simulink model "gm_sampleModel1706_1_sub"  (R2023a)
settings: Solver=VariableStepAuto  StartTime=0.0  StopTime=10.0  RelTol=1e-3
libraries: simulink x4
settings Model: Creator=user1  LastModifiedBy=user1
settings OptimizationCC: BlockReduction=off  ConditionallyExecuteInputs=off
settings DebuggingCC: InheritedTsInSrcMsg=none

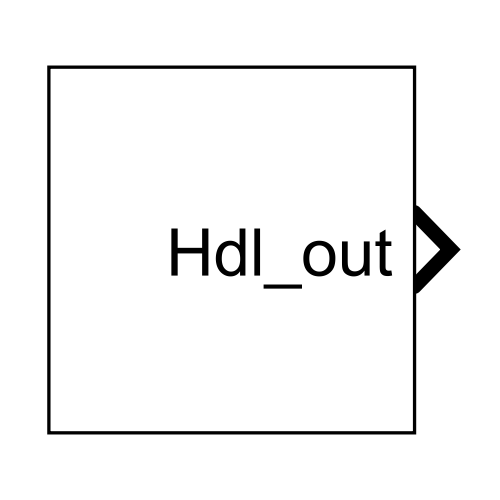
[thumbnail: Simulink's stored preview of the top-level diagram]
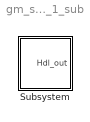
== system gm_sampleModel1706_1_sub ==
  Subsystem : Subsystem

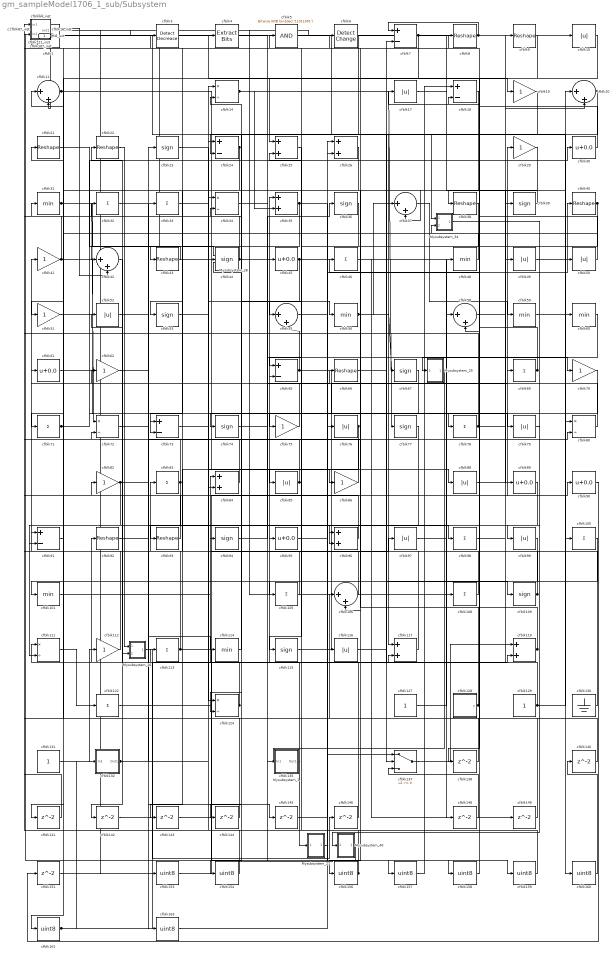
== system gm_sampleModel1706_1_sub/Subsystem ==
  Mysubsystem_1 : Subsystem
  Mysubsystem_25 : Subsystem
  Mysubsystem_26 : Subsystem
  Mysubsystem_27 : Subsystem
  Mysubsystem_28 : Subsystem
  Mysubsystem_34 : Subsystem
  Mysubsystem_40 : Subsystem
  cfblk1 : Logic  AllPortsSameDT=off  OutDataTypeStr=boolean
  cfblk{10,17,49..50,52,76,79,85,88,97,99,116} (12 alike) : Abs  OutDataTypeStr=uint8  SaturateOnIntegerOverflow=off
  cfblk{32..33,46,69,71,78,83,98,100,105,108,113,122} (13 alike) : Sum  Inputs=+  OutDataTypeStr=uint8
  cfblk{31,48,56,59..60,101,114} (7 alike) : MinMax  OutDataTypeStr=uint8
  cfblk103_inst : Subsystem
  cfblk{11,20,37,42,55,58,106} (7 alike) : Sum  Inputs=|++  OutDataTypeStr=uint8
  cfblk107_inst : Subsystem
  cfblk{23,36,39,44,53,67,74,77,94,109,115} (11 alike) : Signum
  cfblk{14,34,72,80,111,124} (6 alike) : Product  Inputs=*/  OutDataTypeStr=uint8  RndMeth=Zero  SaturateOnIntegerOverflow=on
  cfblk{19,29,41,51,62,70,75,82,86,112} (10 alike) : Gain  OutDataTypeStr=uint8
  cfblk{25..26,35,84,96,117,119} (7 alike) : Sum  OutDataTypeStr=uint8
  cfblk121_inst : Subsystem
  cfblk127 : Constant  OutDataTypeStr=uint8  SampleTime=-1
  cfblk128 : Subsystem  mask(Counter Limited){uplimit=double(7), tsamp=double(-1)}
      mask prompts: uplimit "Simulink:masks:UpperLimit_MP"; tsamp "Simulink:masks:SampleTime_MP"
      mask help: Simulink:masks:CounterLimited_MD
      mask init:
      | nbits = double(8);
      | tsamp = double(-1);
      | uplimit = double(7);
  cfblk129 : Constant  OutDataTypeStr=uint8  SampleTime=-1
  cfblk130 : Ground
  cfblk131 : Constant  OutDataTypeStr=uint8  SampleTime=-1
  cfblk132 : Subsystem
  cfblk135 : Subsystem
  cfblk137 : Switch  OutDataTypeStr=uint8  SaturateOnIntegerOverflow=off  InputSameDT=off
  cfblk{138,140..146,148..149,151} (11 alike) : Delay  SampleTime=1
  cfblk{153..154,156..161,163} (9 alike) : DataTypeConversion  OutDataTypeStr=uint8  SaturateOnIntegerOverflow=off  RndMeth=Floor
  cfblk16_inst : Subsystem
  cfblk{7,18,24,65,73,91} (6 alike) : Sum  Inputs=+-  OutDataTypeStr=uint8
  cfblk2 : Constant  Value=0  OutDataTypeStr=uint8  SampleTime=1
  cfblk{8..9,21..22,38,40,43,66,92..93} (10 alike) : Reshape
  cfblk3 : simulink/Logic and Bit Operations/Detect Decrease  vinit=0.0  OutDataTypeStr=uint8
      settings: LibrarySourceBlock=|
      | hdlsllib/Logic and Bit
      | Operations/Detect
      | Decrease
  cfblk{30,45,61,89..90,95} (6 alike) : Bias  Bias=0.0  SaturateOnIntegerOverflow=off
  cfblk4 : simulink/Logic and Bit Operations/Extract Bits  bitsToExtract=Upper half  numBits=8  bitIdxRange=[0 7]  outScalingMode=Preserve fixed-point scaling
      settings: LibrarySourceBlock=|
      | hdlsllib/Logic and Bit
      | Operations/Extract Bits
  cfblk5 : simulink/Logic and Bit Operations/Bitwise Operator  logicop=AND  UseBitMask=on  BitMask=bin2dec('11011001')  BitMaskRealWorld=Stored Integer
      settings: LibrarySourceBlock=|
      | hdlsllib/Logic and Bit
      | Operations/Bitwise
      | Operator
  cfblk6 : simulink/Logic and Bit Operations/Detect Change  vinit=0  OutDataTypeStr=uint8
      settings: LibrarySourceBlock=|
      | hdlsllib/Logic and Bit
      | Operations/Detect
      | Change
  cfblk64_inst : Subsystem
  cfblk87_inst : Subsystem
  Hdl_out : Outport  OutDataTypeStr=uint8  SampleTime=1
  wires:
  Mysubsystem_1/1(Out1) -> Mysubsystem_27/1(In1)
  Mysubsystem_25/1(Out1) -> Mysubsystem_1/1(In1)
  Mysubsystem_26/1(Out1) -> cfblk146/1
  Mysubsystem_27/1(Out1) -> cfblk26/1
  Mysubsystem_28/1(Out1) -> cfblk149/1
  Mysubsystem_34/1(Out1) -> Mysubsystem_40/1(In1)
  Mysubsystem_40/1(Out1) -> cfblk64_inst/2(in2)
  cfblk1/1 -> cfblk117/1
  cfblk10/1 -> cfblk25/1
  cfblk100/1 -> cfblk101/1
  cfblk101/1 -> cfblk84/1
  cfblk103_inst/1(out1) -> cfblk4/1
  cfblk105/1 -> cfblk35/1
  cfblk106/1 -> cfblk41/1
  cfblk107_inst/1(out1) -> cfblk45/1, cfblk33/1
  cfblk108/1 -> cfblk103_inst/1(in1)
  cfblk109/1 -> cfblk58/2, Mysubsystem_28/2(In2)
  cfblk11/1 -> cfblk88/1, cfblk71/1
  cfblk111/1 -> cfblk122/1
  cfblk112/1 -> cfblk121_inst/1(in1)
  cfblk113/1 -> cfblk91/1, cfblk158/1, cfblk29/1
  cfblk114/1 -> cfblk34/2
  cfblk115/1 -> cfblk69/1
  cfblk116/1 -> cfblk90/1
  cfblk117/1 -> cfblk3/1
  cfblk119/1 -> cfblk38/1, cfblk103_inst/2(in2)
  cfblk121_inst/1(out1) -> cfblk10/1
  cfblk122/1 -> cfblk97/1
  cfblk124/1 -> cfblk92/1, cfblk22/1
  cfblk127/1 -> cfblk58/1
  cfblk128/1(y) -> cfblk72/2, cfblk113/1
  cfblk129/1 -> cfblk20/1, cfblk111/1
  cfblk130/1 -> cfblk83/1
  cfblk131/1 -> cfblk112/1
  cfblk132/1(Out1) -> cfblk44/1, cfblk23/1
  cfblk135/1(Out1) -> cfblk94/1
  cfblk137/1 -> cfblk119/1
  cfblk138/1 -> cfblk1/1
  cfblk14/1 -> cfblk77/1, cfblk35/2
  cfblk140/1 -> cfblk107_inst/1(in1)
  cfblk141/1 -> cfblk87_inst/1(in1)
  cfblk142/1 -> cfblk7/2
  cfblk143/1 -> cfblk117/2
  cfblk144/1 -> cfblk1/2
  cfblk145/1 -> cfblk137/1
  cfblk146/1 -> cfblk65/2
  cfblk148/1 -> cfblk137/3
  cfblk149/1 -> cfblk106/1
  cfblk151/1 -> cfblk119/2
  cfblk153/1 -> cfblk95/1
  cfblk154/1 -> cfblk64_inst/1(in1)
  cfblk156/1 -> cfblk87_inst/2(in2), cfblk34/1
  cfblk157/1 -> cfblk18/1
  cfblk158/1 -> cfblk18/2
  cfblk159/1 -> cfblk5/1
  cfblk16_inst/1(out1) -> cfblk108/1
  cfblk160/1 -> cfblk140/1
  cfblk161/1 -> cfblk9/1, cfblk132/1(In1)
  cfblk163/1 -> cfblk26/2
  cfblk17/1 -> cfblk100/1
  cfblk18/1 -> cfblk156/1
  cfblk19/1 -> cfblk137/2
  cfblk2/1 -> cfblk42/2
  cfblk20/1 -> cfblk24/2, Mysubsystem_34/1(In1)
  cfblk21/1 -> cfblk43/1
  cfblk22/1 -> Mysubsystem_26/1(In1)
  cfblk23/1 -> cfblk86/1
  cfblk24/1 -> cfblk53/1, cfblk141/1
  cfblk25/1 -> cfblk85/1
  cfblk26/1 -> cfblk161/1
  cfblk29/1 -> cfblk84/2
  cfblk3/1 -> cfblk19/1
  cfblk30/1 -> cfblk8/1
  cfblk31/1 -> cfblk72/1, Mysubsystem_28/1(In1)
  cfblk32/1 -> cfblk96/2
  cfblk33/1 -> cfblk56/1
  cfblk34/1 -> cfblk159/1
  cfblk35/1 -> cfblk76/1, cfblk73/2
  cfblk36/1 -> cfblk55/1
  cfblk37/1 -> cfblk59/1
  cfblk38/1 -> cfblk65/1
  cfblk39/1 -> cfblk37/2
  cfblk4/1 -> cfblk96/1
  cfblk40/1 -> cfblk75/1, Mysubsystem_34/2(In2)
  cfblk41/1 -> cfblk135/1(In1), cfblk31/1
  cfblk42/1 -> cfblk142/1
  cfblk43/1 -> cfblk42/1
  cfblk44/1 -> cfblk107_inst/2(in2), cfblk70/1
  cfblk45/1 -> cfblk25/2, cfblk124/2
  cfblk46/1 -> cfblk148/1
  cfblk48/1 -> cfblk11/1
  cfblk49/1 -> cfblk40/1
  cfblk5/1 -> cfblk160/1
  cfblk50/1 -> cfblk17/1
  cfblk51/1 -> cfblk78/1
  cfblk52/1 -> cfblk114/1
  cfblk53/1 -> cfblk14/1
  cfblk55/1 -> cfblk50/1
  cfblk56/1 -> cfblk67/1, cfblk37/1
  cfblk58/1 -> cfblk20/2
  cfblk59/1 -> cfblk60/1
  cfblk6/1 -> cfblk154/1
  cfblk60/1 -> Mysubsystem_25/1(In1)
  cfblk61/1 -> cfblk116/1
  cfblk62/1 -> cfblk163/1
  cfblk64_inst/1(out1) -> cfblk153/1
  cfblk65/1 -> cfblk79/1, cfblk55/2
  cfblk66/1 -> cfblk109/1
  cfblk67/1 -> cfblk115/1
  cfblk69/1 -> cfblk6/1, cfblk46/1
  cfblk7/1 -> cfblk89/1, cfblk51/1
  cfblk70/1 -> cfblk74/1
  cfblk71/1 -> cfblk73/1, cfblk30/1
  cfblk72/1 -> cfblk98/1
  cfblk73/1 -> cfblk124/1
  cfblk74/1 -> cfblk66/1
  cfblk75/1 -> cfblk24/1
  cfblk76/1 -> cfblk144/1, cfblk143/1
  cfblk77/1 -> cfblk91/2
  cfblk78/1 -> cfblk49/1, cfblk16_inst/1(in1), cfblk14/2
  cfblk79/1 -> cfblk99/1
  cfblk8/1 -> cfblk7/1, Hdl_out/1
  cfblk80/1 -> cfblk61/1
  cfblk82/1 -> cfblk80/2, cfblk111/2
  cfblk83/1 -> cfblk93/1, cfblk16_inst/2(in2)
  cfblk84/1 -> cfblk62/1
  cfblk85/1 -> cfblk52/1, cfblk105/1
  cfblk86/1 -> cfblk32/1
  cfblk87_inst/1(out1) -> cfblk11/2
  cfblk88/1 -> cfblk39/1
  cfblk89/1 -> Mysubsystem_26/2(In2)
  cfblk9/1 -> cfblk138/1
  cfblk90/1 -> cfblk151/1
  cfblk91/1 -> cfblk21/1
  cfblk92/1 -> cfblk145/1
  cfblk93/1 -> cfblk82/1
  cfblk94/1 -> cfblk36/1
  cfblk95/1 -> cfblk157/1
  cfblk96/1 -> cfblk121_inst/2(in2)
  cfblk97/1 -> cfblk48/1
  cfblk98/1 -> cfblk80/1
  cfblk99/1 -> cfblk106/2

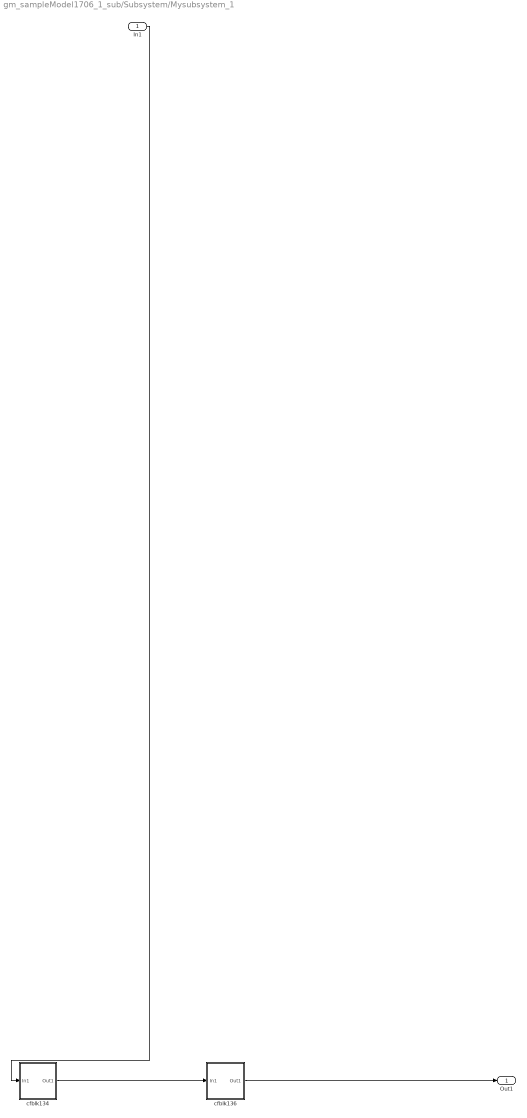
== system gm_sampleModel1706_1_sub/Subsystem/Mysubsystem_1 ==
  In1 : Inport  OutDataTypeStr=uint8  PortDimensions=1  SampleTime=1
  cfblk134 : Subsystem
  cfblk136 : Subsystem
  Out1 : Outport  SampleTime=1
  wires:
  In1/1 -> cfblk134/1(In1)
  cfblk134/1(Out1) -> cfblk136/1(In1)
  cfblk136/1(Out1) -> Out1/1

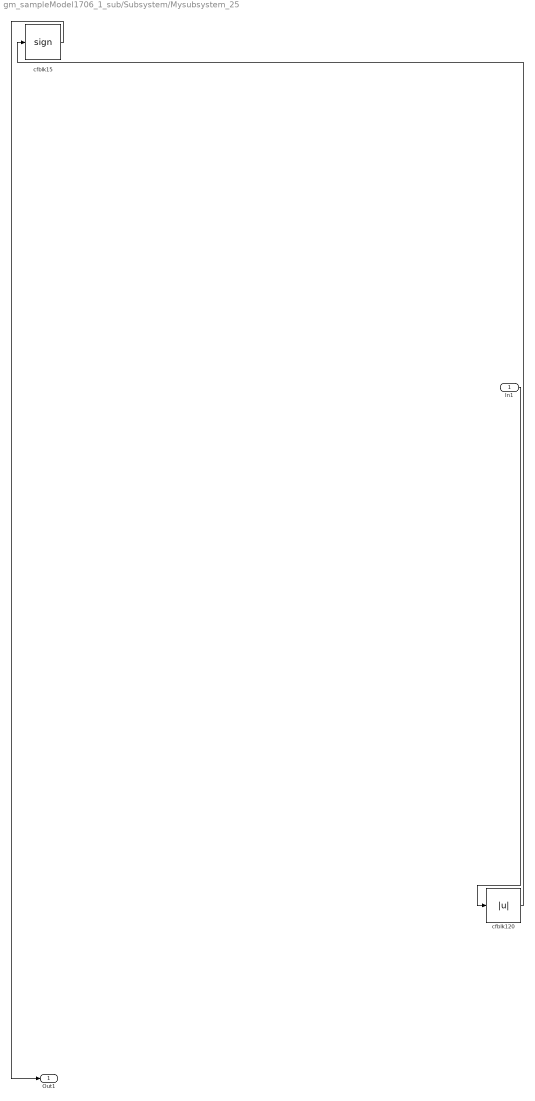
== system gm_sampleModel1706_1_sub/Subsystem/Mysubsystem_25 ==
  In1 : Inport  OutDataTypeStr=uint8  PortDimensions=1  SampleTime=1
  cfblk120 : Abs  SaturateOnIntegerOverflow=off
  cfblk15 : Signum
  Out1 : Outport  SampleTime=1
  wires:
  In1/1 -> cfblk120/1
  cfblk120/1 -> cfblk15/1
  cfblk15/1 -> Out1/1

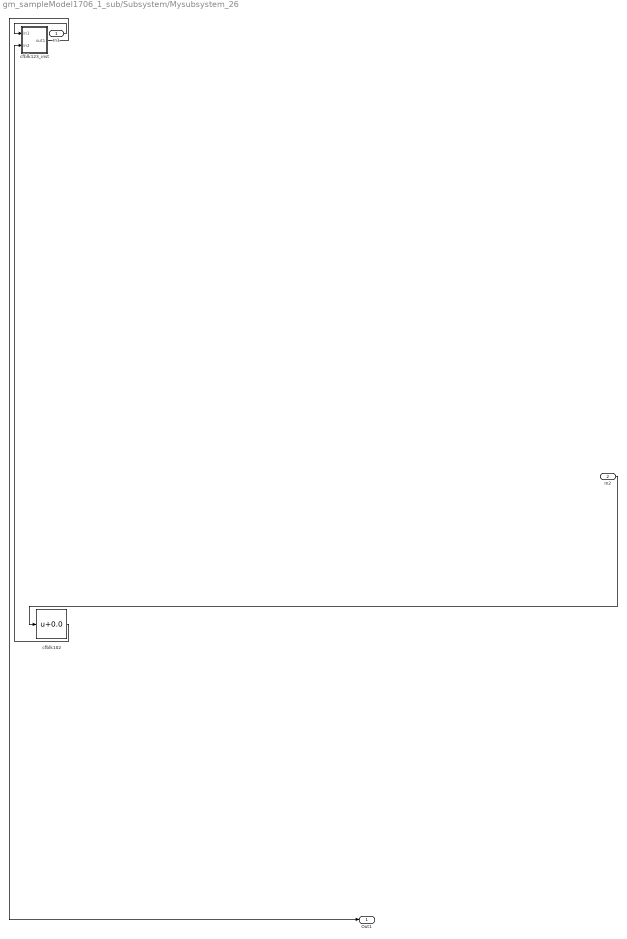
== system gm_sampleModel1706_1_sub/Subsystem/Mysubsystem_26 ==
  In1 : Inport  OutDataTypeStr=uint8  PortDimensions=1  SampleTime=1
  In2 : Inport  Port=2  OutDataTypeStr=uint8  PortDimensions=1  SampleTime=1
  cfblk102 : Bias  Bias=0.0  SaturateOnIntegerOverflow=off
  cfblk123_inst : Subsystem
  Out1 : Outport  SampleTime=1
  wires:
  In1/1 -> cfblk123_inst/1(in1)
  In2/1 -> cfblk102/1
  cfblk102/1 -> cfblk123_inst/2(in2)
  cfblk123_inst/1(out1) -> Out1/1

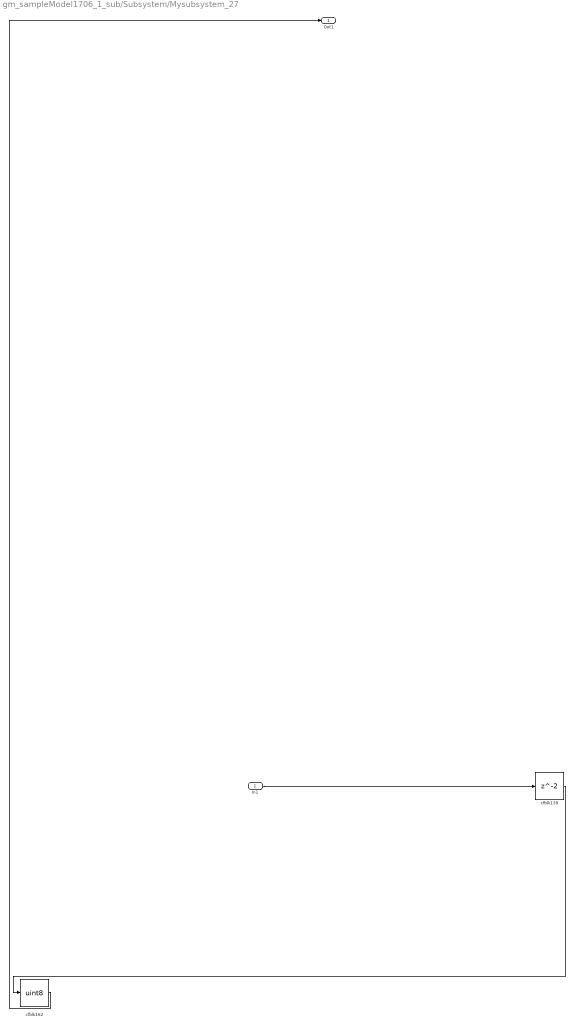
== system gm_sampleModel1706_1_sub/Subsystem/Mysubsystem_27 ==
  In1 : Inport  OutDataTypeStr=uint8  PortDimensions=1  SampleTime=1
  cfblk139 : Delay  SampleTime=1
  cfblk162 : DataTypeConversion  OutDataTypeStr=uint8  SaturateOnIntegerOverflow=off  RndMeth=Floor
  Out1 : Outport  SampleTime=1
  wires:
  In1/1 -> cfblk139/1
  cfblk139/1 -> cfblk162/1
  cfblk162/1 -> Out1/1

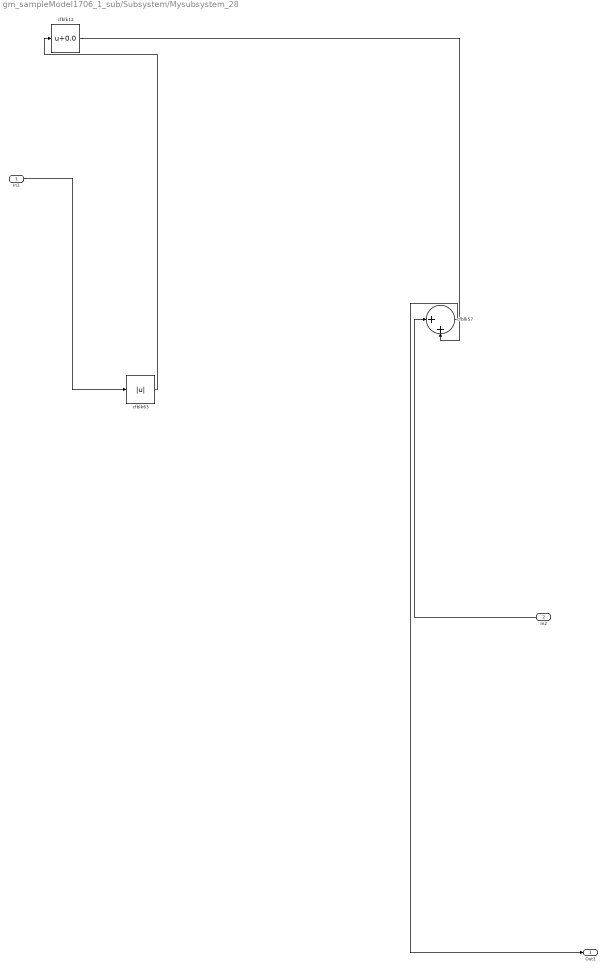
== system gm_sampleModel1706_1_sub/Subsystem/Mysubsystem_28 ==
  In1 : Inport  OutDataTypeStr=uint8  PortDimensions=1  SampleTime=1
  In2 : Inport  Port=2  OutDataTypeStr=uint8  PortDimensions=1  SampleTime=1
  cfblk12 : Bias  Bias=0.0  SaturateOnIntegerOverflow=off
  cfblk57 : Sum  Inputs=|++
  cfblk63 : Abs  SaturateOnIntegerOverflow=off
  Out1 : Outport  SampleTime=1
  wires:
  In1/1 -> cfblk63/1
  In2/1 -> cfblk57/1
  cfblk12/1 -> cfblk57/2
  cfblk57/1 -> Out1/1
  cfblk63/1 -> cfblk12/1

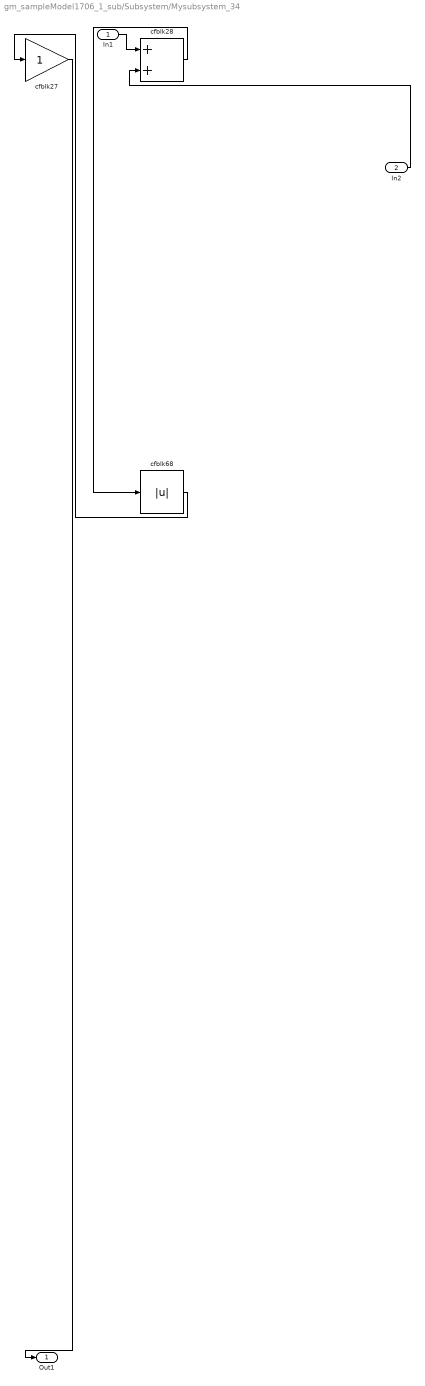
== system gm_sampleModel1706_1_sub/Subsystem/Mysubsystem_34 ==
  In1 : Inport  OutDataTypeStr=uint8  PortDimensions=1  SampleTime=1
  In2 : Inport  Port=2  OutDataTypeStr=uint8  PortDimensions=1  SampleTime=1
  cfblk27 : Gain
  cfblk28 : Sum
  cfblk68 : Abs  SaturateOnIntegerOverflow=off
  Out1 : Outport  SampleTime=1
  wires:
  In1/1 -> cfblk28/1
  In2/1 -> cfblk28/2
  cfblk27/1 -> Out1/1
  cfblk28/1 -> cfblk68/1
  cfblk68/1 -> cfblk27/1

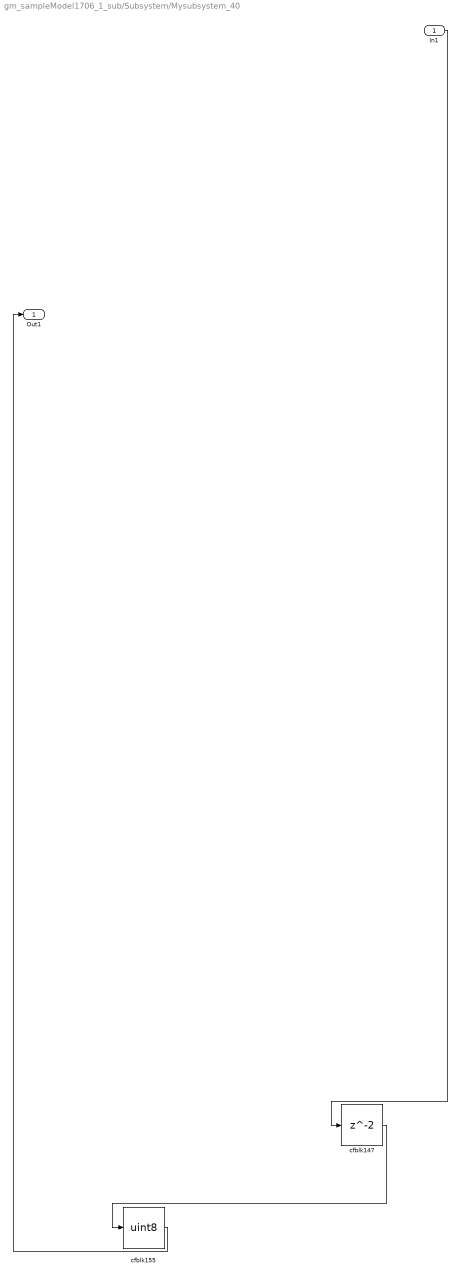
== system gm_sampleModel1706_1_sub/Subsystem/Mysubsystem_40 ==
  In1 : Inport  OutDataTypeStr=fixdt(0, 16, 7)  PortDimensions=1  SampleTime=1
  cfblk147 : Delay  SampleTime=1
  cfblk155 : DataTypeConversion  OutDataTypeStr=uint8  SaturateOnIntegerOverflow=off  RndMeth=Floor
  Out1 : Outport  SampleTime=1
  wires:
  In1/1 -> cfblk147/1
  cfblk147/1 -> cfblk155/1
  cfblk155/1 -> Out1/1

== system gm_sampleModel1706_1_sub/Subsystem/cfblk103_inst ==
  in1 : Inport  OutDataTypeStr=uint8  SampleTime=1
  in2 : Inport  Port=2  OutDataTypeStr=uint8  SampleTime=1
  mul_cfblk103_dotp_mulcomp : Product  Inputs=**  OutDataTypeStr=uint8  SampleTime=1
  out1 : Outport  OutDataTypeStr=uint8  SampleTime=1
  wires:
  in1/1 -> mul_cfblk103_dotp_mulcomp/1
  in2/1 -> mul_cfblk103_dotp_mulcomp/2
  mul_cfblk103_dotp_mulcomp/1 -> out1/1

== system gm_sampleModel1706_1_sub/Subsystem/cfblk107_inst ==
  in1 : Inport  OutDataTypeStr=uint8  SampleTime=1
  in2 : Inport  Port=2  OutDataTypeStr=uint8  SampleTime=1
  mul_cfblk107_dotp_mulcomp : Product  Inputs=**  OutDataTypeStr=uint8  SampleTime=1
  out1 : Outport  OutDataTypeStr=uint8  SampleTime=1
  wires:
  in1/1 -> mul_cfblk107_dotp_mulcomp/1
  in2/1 -> mul_cfblk107_dotp_mulcomp/2
  mul_cfblk107_dotp_mulcomp/1 -> out1/1

== system gm_sampleModel1706_1_sub/Subsystem/cfblk121_inst ==
  in1 : Inport  OutDataTypeStr=uint8  SampleTime=1
  in2 : Inport  Port=2  OutDataTypeStr=uint8  SampleTime=1
  mul_cfblk121_dotp_mulcomp : Product  Inputs=**  OutDataTypeStr=uint8  SampleTime=1
  out1 : Outport  OutDataTypeStr=uint8  SampleTime=1
  wires:
  in1/1 -> mul_cfblk121_dotp_mulcomp/1
  in2/1 -> mul_cfblk121_dotp_mulcomp/2
  mul_cfblk121_dotp_mulcomp/1 -> out1/1

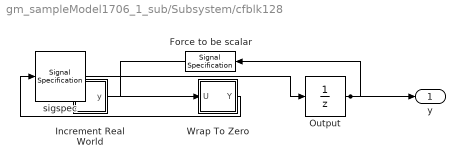
== system gm_sampleModel1706_1_sub/Subsystem/cfblk128 ==
  Force to be scalar : SignalSpecification  DisableCoverage=on  Dimensions=1
  Increment Real World : Subsystem  mask(Real World Value Increment){}
      mask help: Simulink:masks:RealWorldValueIncrement_MD
      mask Display: disp('V++')
  Output : UnitDelay  InitialCondition=0.0  SampleTime=tsamp  HasFrameUpgradeWarning=on
  Wrap To Zero : Subsystem  mask(Wrap To Zero){Threshold=double(7)}
      mask prompts: Threshold "Simulink:masks:Threshold_MP"
      mask help: Simulink:masks:WrapToZero_MD
  sigspec : SignalSpecification  OutDataTypeStr=uint8  Dimensions=1
  y : Outport  SampleTime=1
  wires:
  Force to be scalar/1 -> Increment Real World/1(u)
  Increment Real World/1(y) -> Wrap To Zero/1(U)
  Output/1 -> Force to be scalar/1, y/1
  Wrap To Zero/1(Y) -> sigspec/1
  sigspec/1 -> Output/1

== system gm_sampleModel1706_1_sub/Subsystem/cfblk132 ==
  In1 : Inport  OutDataTypeStr=uint8  PortDimensions=1  SampleTime=1
  Out1 : Outport  SampleTime=1
  wires:
  In1/1 -> Out1/1

== system gm_sampleModel1706_1_sub/Subsystem/cfblk135 ==
  In1 : Inport  OutDataTypeStr=uint8  PortDimensions=1  SampleTime=1
  Out1 : Outport  SampleTime=1
  wires:
  In1/1 -> Out1/1

== system gm_sampleModel1706_1_sub/Subsystem/cfblk16_inst ==
  in1 : Inport  OutDataTypeStr=uint8  SampleTime=1
  in2 : Inport  Port=2  OutDataTypeStr=uint8  SampleTime=1
  mul_cfblk16_dotp_mulcomp : Product  Inputs=**  OutDataTypeStr=uint8  SampleTime=1
  out1 : Outport  OutDataTypeStr=uint8  SampleTime=1
  wires:
  in1/1 -> mul_cfblk16_dotp_mulcomp/1
  in2/1 -> mul_cfblk16_dotp_mulcomp/2
  mul_cfblk16_dotp_mulcomp/1 -> out1/1

== system gm_sampleModel1706_1_sub/Subsystem/cfblk64_inst ==
  in1 : Inport  OutDataTypeStr=uint8  SampleTime=1
  in2 : Inport  Port=2  OutDataTypeStr=uint8  SampleTime=1
  mul_cfblk64_dotp_mulcomp : Product  Inputs=**  OutDataTypeStr=uint8  SampleTime=1
  out1 : Outport  OutDataTypeStr=uint8  SampleTime=1
  wires:
  in1/1 -> mul_cfblk64_dotp_mulcomp/1
  in2/1 -> mul_cfblk64_dotp_mulcomp/2
  mul_cfblk64_dotp_mulcomp/1 -> out1/1

== system gm_sampleModel1706_1_sub/Subsystem/cfblk87_inst ==
  in1 : Inport  OutDataTypeStr=uint8  SampleTime=1
  in2 : Inport  Port=2  OutDataTypeStr=uint8  SampleTime=1
  mul_cfblk87_dotp_mulcomp : Product  Inputs=**  OutDataTypeStr=uint8  SampleTime=1
  out1 : Outport  OutDataTypeStr=uint8  SampleTime=1
  wires:
  in1/1 -> mul_cfblk87_dotp_mulcomp/1
  in2/1 -> mul_cfblk87_dotp_mulcomp/2
  mul_cfblk87_dotp_mulcomp/1 -> out1/1

== system gm_sampleModel1706_1_sub/Subsystem/Mysubsystem_1/cfblk134 ==
  In1 : Inport  OutDataTypeStr=uint8  PortDimensions=1  SampleTime=1
  Out1 : Outport  SampleTime=1
  wires:
  In1/1 -> Out1/1

== system gm_sampleModel1706_1_sub/Subsystem/Mysubsystem_1/cfblk136 ==
  In1 : Inport  OutDataTypeStr=uint8  PortDimensions=1  SampleTime=1
  Out1 : Outport  SampleTime=1
  wires:
  In1/1 -> Out1/1

== system gm_sampleModel1706_1_sub/Subsystem/Mysubsystem_26/cfblk123_inst ==
  in1 : Inport  OutDataTypeStr=uint8  SampleTime=1
  in2 : Inport  Port=2  OutDataTypeStr=uint8  SampleTime=1
  mul_cfblk123_dotp_mulcomp : Product  Inputs=**  OutDataTypeStr=uint16  SampleTime=1
  out1 : Outport  OutDataTypeStr=uint16  SampleTime=1
  wires:
  in1/1 -> mul_cfblk123_dotp_mulcomp/1
  in2/1 -> mul_cfblk123_dotp_mulcomp/2
  mul_cfblk123_dotp_mulcomp/1 -> out1/1

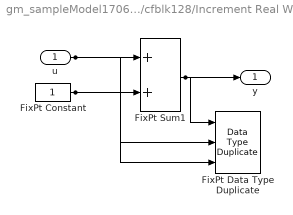
== system gm_sampleModel1706_1_sub/Subsystem/cfblk128/Increment Real World ==
  u : Inport  OutDataTypeStr=uint8  SampleTime=1
  FixPt Constant : Constant  DisableCoverage=on  OutDataTypeStr=Inherit: Inherit via back propagation  SampleTime=-1
  FixPt Data Type Duplicate : DataTypeDuplicate  DisableCoverage=on  NumInputPorts=3
  FixPt Sum1 : Sum  InputSameDT=on  OutDataTypeStr=Inherit: Inherit via back propagation  LockScale=on
  y : Outport  SampleTime=1
  wires:
  u/1 -> FixPt Sum1/1, FixPt Data Type Duplicate/2
  FixPt Constant/1 -> FixPt Sum1/2, FixPt Data Type Duplicate/3
  FixPt Sum1/1 -> FixPt Data Type Duplicate/1, y/1

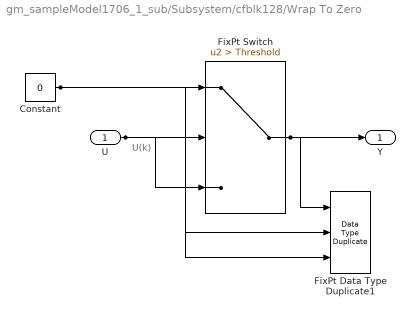
== system gm_sampleModel1706_1_sub/Subsystem/cfblk128/Wrap To Zero ==
  note: U(k)
  U : Inport  OutDataTypeStr=uint8  SampleTime=1
  Constant : Constant  DisableCoverage=on  Value=0  OutDataTypeStr=Inherit: Inherit via back propagation  SampleTime=-1
  FixPt Data Type Duplicate1 : DataTypeDuplicate  DisableCoverage=on  NumInputPorts=3
  FixPt Switch : Switch  Criteria=u2 > Threshold  Threshold=Threshold  OutDataTypeStr=Inherit: Inherit via back propagation  ZeroCross=off  SaturateOnIntegerOverflow=off  InputSameDT=off
  Y : Outport  SampleTime=1
  wires:
  U/1 -> FixPt Switch/3, FixPt Switch/2, FixPt Data Type Duplicate1/2
  Constant/1 -> FixPt Switch/1, FixPt Data Type Duplicate1/3
  FixPt Switch/1 -> FixPt Data Type Duplicate1/1, Y/1
